simulink model "valve_ports"  (R2020b)
settings: Solver=VariableStepAuto  StartTime=0.0  StopTime=inf  RelTol=1e-3
undefined symbols (not defined in the file): daq
libraries: daqlib x2, eeGeneralControl x1
settings Model: Creator=SIRIL D. TEJA  LastModifiedBy=SIRIL D. TEJA

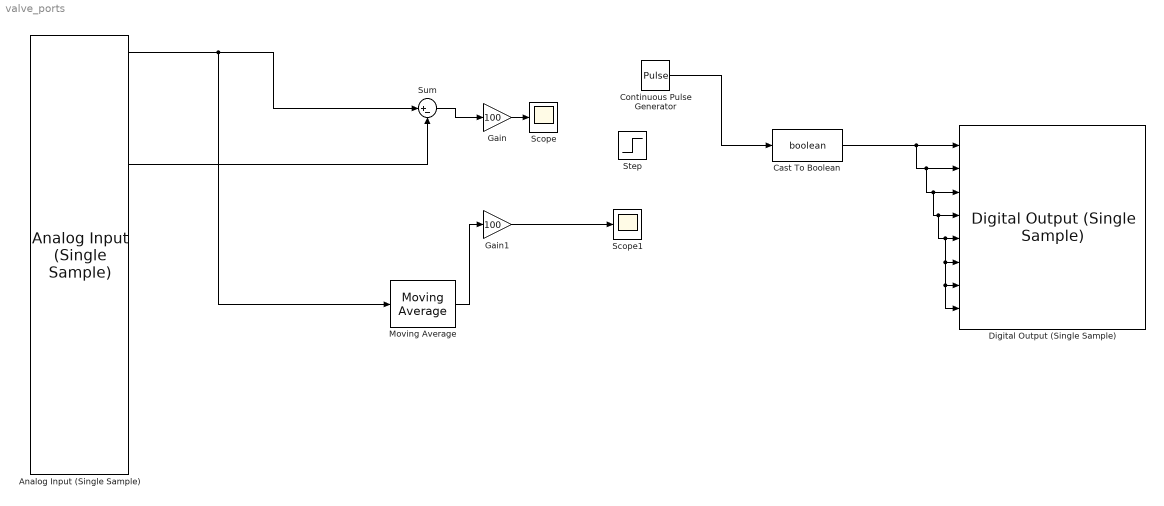
== system valve_ports ==
  Analog Input (Single Sample) : daqlib/Analog Input (Single Sample)  DeviceMenu=ni cDAQ1 (cDAQ-9178)  Device=ni cDAQ1 (cDAQ-9178)  ModuleInfo=cDAQ1Mod5(NI 9205)  ObjConstructor=daq.createSession('ni')  BlockSampleTime=1  NChannelsSelected=32  Channels=1$ai0$$cDAQ1Mod5$1$4$3$1$#1$ai1$$cDAQ1Mod5$1$4$3$1$#1$ai2$$cDAQ1Mod5$1$4$3$1$#1$ai3$$cDAQ1Mod5$1$4$3$1$#1$ai4$$cDAQ1Mod5$1$4$3$1$#1$ai5$$cDAQ1Mod5$1$4$3$1$#1$ai6$$cDAQ1Mod5$1$4$3$1$#1$ai7$$cDAQ1Mod5$1$4$3$1$#1$ai8$$cDAQ1Mod5$1$4$1$1$#1$ai9$$cDAQ1Mod5$1$4$1$1$#1$ai10$$cDAQ1Mod5$1$4$1$1$#1$ai11$$cDAQ1Mod5$1$4$1$1$#1$ai12$$cDAQ1Mod5$1$4$1$1$#1$ai13$$cDAQ1Mod5$1$4$1$1$#1$ai14$$cDAQ1Mod5$1$4$1$1$#1$ai15$$cDAQ1Mod5$1$4$1$1$#1$ai16$$cDAQ1Mod5$1$4$3$1$#1$ai17$$cDAQ1Mod5$1$4$3$1$#1$ai18$$cDAQ1Mod5$1$4$3$1$#1$ai19$$cDAQ1Mod5$1$4$3$1$#1$ai20$$cDAQ1Mod5$1$4$3$1$#1$ai21$$cDAQ1Mod5$1$4$3$1$#1$ai22$$cDAQ1Mod5$1$4$3$1$#1$ai23$$cDAQ1Mod5$1$4$3$1$#1$ai24$$cDAQ1Mod5$1$4$1$1$#1$ai25$$cDAQ1Mod5$1$4$1$1$#1$ai26$$cDAQ1Mod5$1$4$1$1$#1$ai27$$cDAQ1Mod5$1$4$1$1$#1$ai28$$cDAQ1Mod5$1$4$1$1$#1$ai29$$cDAQ1Mod5$1$4$1$1$#1$ai30$$cDAQ1Mod5$1$4$1$1$#1$ai31$$cDAQ1Mod5$1$4$1$1$#  NPorts=1 per channel  OutputTimestamp=off
      settings: SourceProductBaseCode=DA
  Cast To Boolean : DataTypeConversion  OutDataTypeStr=boolean
  Continuous Pulse Generator : DiscretePulseGenerator  PulseType=Time based  Period=50  PulseWidth=50  PhaseDelay=1
  Digital Output (Single Sample) : daqlib/Digital Output (Single Sample)  DeviceMenu=ni cDAQ1 (cDAQ-9178)  Device=ni cDAQ1 (cDAQ-9178)  ModuleInfo=cDAQ1Mod1(NI 9485)  ObjConstructor=daq.createSession('ni')  BlockSampleTime=1  IsDigitalInput=off  NLinesSelected=8  Lines=1$port0/line0$$cDAQ1Mod1$#1$port0/line1$$cDAQ1Mod1$#1$port0/line2$$cDAQ1Mod1$#1$port0/line3$$cDAQ1Mod1$#1$port0/line4$$cDAQ1Mod1$#1$port0/line5$$cDAQ1Mod1$#1$port0/line6$$cDAQ1Mod1$#1$port0/line7$$cDAQ1Mod1$#  NPorts=1 per line
      settings: SourceProductBaseCode=DA
  Gain : Gain  Gain=100
  Gain1 : Gain  Gain=100
  Moving Average : eeGeneralControl/Moving Average  VariantControl=Variant1  LabelModeActiveChoice=Discrete  f=60  x0=0  Ts=-1
      settings: SourceProductBaseCode=PS
  Scope : Scope
  Scope1 : Scope
  Step : Step  OutDataTypeStr=Inherit: Inherit via back propagation  SampleTime=0
  Sum : Sum  Inputs=|+-
  wires:
  Cast To Boolean/1 -> Digital Output (Single Sample)/8, Digital Output (Single Sample)/7, Digital Output (Single Sample)/6, Digital Output (Single Sample)/5, Digital Output (Single Sample)/4, Digital Output (Single Sample)/3, Digital Output (Single Sample)/2, Digital Output (Single Sample)/1
  Continuous Pulse Generator/1 -> Cast To Boolean/1
  Analog Input (Single Sample)/10 -> Sum/2
  Gain/1 -> Scope/1
  Sum/1 -> Gain/1
  Analog Input (Single Sample)/2 -> Moving Average/1, Sum/1
  Gain1/1 -> Scope1/1
  Moving Average/1 -> Gain1/1
